simulink model "kont_lqr_pid"  (R2022b)
settings: Solver=VariableStepAuto  StartTime=0.0  StopTime=5  RelTol=1e-3
values from neighbouring files (symbols this model uses):
  A = [0    -g   0    0    0    0    0    0 ... (first row only)    [fDOF_sim_V2.m]
  B = [0          g       0 ... (first row only)    [fDOF_sim_V2.m]
undefined symbols (not defined in the file or in its folder): DiscIntNeverNeededParam, Kd
settings Model: Creator=Edvin  LastModifiedBy=Edvin

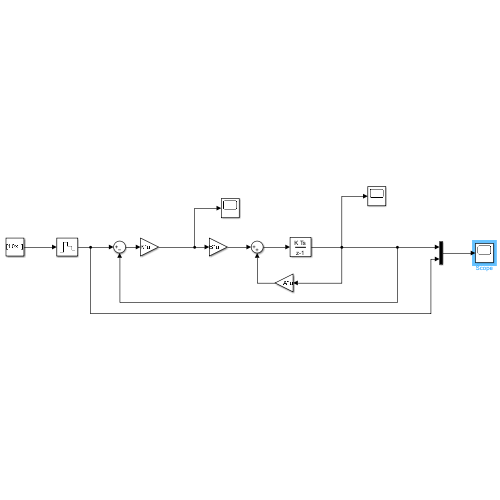
[thumbnail: Simulink's stored preview of the top-level diagram]
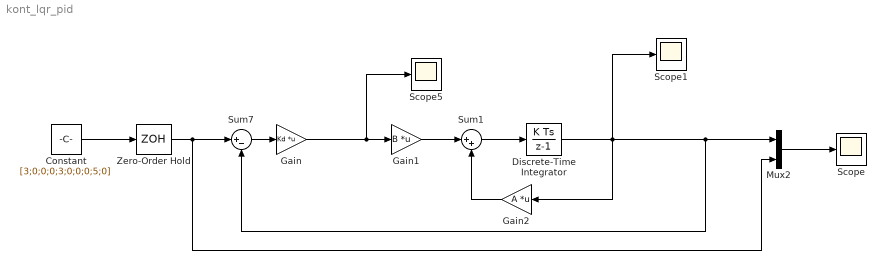
== system kont_lqr_pid ==
  Constant : Constant  Value=[3;0;0;0;3;0;0;0;5;0]
  Discrete-Time Integrator : DiscreteIntegrator  SampleTime=-1  ICPrevOutput=DiscIntNeverNeededParam  ICPrevScaledInput=DiscIntNeverNeededParam
  Gain : Gain  Gain=Kd  Multiplication=Matrix(K*u)
  Gain1 : Gain  Gain=B  Multiplication=Matrix(K*u)
  Gain2 : Gain  Gain=A  Multiplication=Matrix(K*u)
  Mux2 : Mux  Inputs=2
  Scope : Scope
  Scope1 : Scope
  Scope5 : Scope
  Sum1 : Sum  Inputs=|++
  Sum7 : Sum  Inputs=|+-
  Zero-Order Hold : ZeroOrderHold  SampleTime=0.01
  wires:
  Gain1/1 -> Sum1/1
  Sum1/1 -> Discrete-Time Integrator/1
  Gain2/1 -> Sum1/2
  Sum7/1 -> Gain/1
  Constant/1 -> Zero-Order Hold/1
  Mux2/1 -> Scope/1
  Gain/1 -> Scope5/1, Gain1/1
  Discrete-Time Integrator/1 -> Mux2/1, Sum7/2, Scope1/1, Gain2/1
  Zero-Order Hold/1 -> Mux2/2, Sum7/1
